simulink library "roller485lib"  (R2023a)
settings: Solver=VariableStepAuto  StartTime=0.0  StopTime=10.0  RelTol=1e-3
libraries: arduinolib x173, simulink x66
(part 1 of 6)
settings Model: Creator=kawata  LastModifiedBy=kawata
settings RTWCC: GPUComputeCapability=5.0

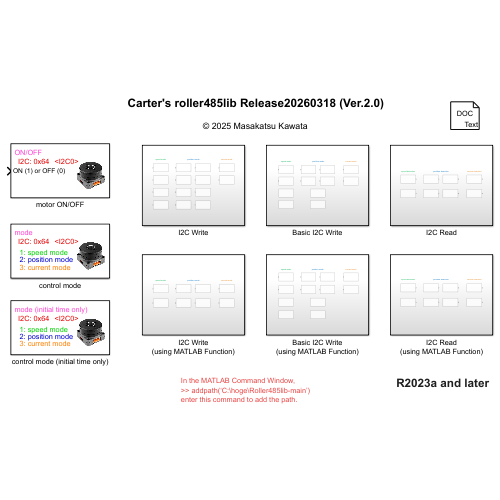
[thumbnail: Simulink's stored preview of the top-level diagram]
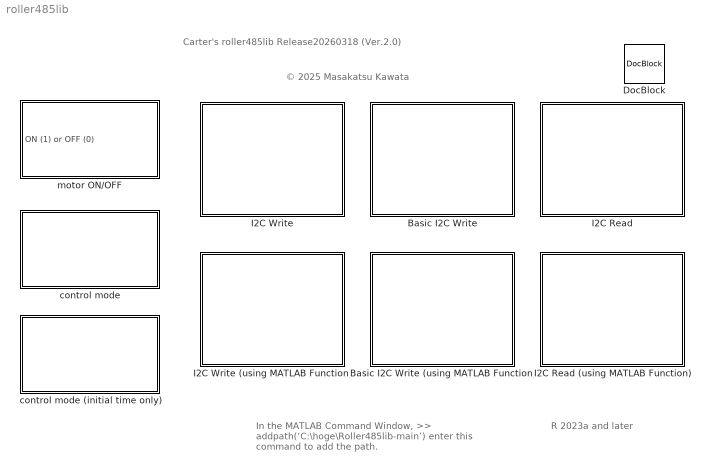
== system roller485lib ==
  note: © 2025 Masakatsu Kawata
  note: Carter's roller485lib Release20260318 (Ver.2.0)
  note: R 2023a and later
  note: In the MATLAB Command Window,
      | >> addpath(‘C:\hoge\Roller485lib-main’)
      | enter this command to add the path.
  Basic I2C Write : Subsystem
  Basic I2C Write (using MATLAB Function) : Subsystem
  DocBlock : simulink/Model-Wide Utilities/DocBlock  DocumentType=Text
      content=|
      | Carter's Roller485lib Ver.1.0
      | Copyright (c) 2025 Masakatsu Kawata
      | Released under the MIT License.
      | See LICENSE for details.
  I2C Read : Subsystem
  I2C Read (using MATLAB Function) : Subsystem
  I2C Write : Subsystem
  I2C Write (using MATLAB Function) : Subsystem
  control mode : Subsystem  mask{I2CAddress=0x64, I2CModule=0, control_mode=1}
      mask prompts: I2CAddress "I2C Address"; I2CModule "I2C Module"; control_mode "mode"
      mask help:
      | 1: speed mode (default)
      | 2: position mode
      | 3: current mode
      | 4: encoder mode
      mask TypeOptions I2CModule:
      | I2C Write
      | (0x01)/I2CModule
      mask DialogControl ParameterGroupVar Prompt: パラメーター
      mask Display:
      | image('roller485.png', [55,10,75,56]);
      | color('magenta');
      | text(5, 62, 'mode');
      | color('green');
      | text(12, 35, '1: speed mode');
      | color('blue');
      | text(12, 25, '2: position mode');
      | color('orange');
      | text(12, 15, '3: current mode');
      | 
      | color('red');
      | addr = get_param(gcb, 'I2CAddress');
      | text(10, 50, ['I2C: ' addr]);
      | 
      | color('red');
      | module = get_param(gcb, 'I2CModule');
      | text(60, 50, ['<I2C' module '>']);
  control mode (initial time only) : Subsystem  mask{I2CAddress=0x64, I2CModule=0, control_mode=1}
      mask prompts: I2CAddress "I2C Address"; I2CModule "I2C Module"; control_mode "mode"
      mask help:
      | 1: speed mode (default)
      | 2: position mode
      | 3: current mode
      | 4: encoder mode
      | ---------------------------------
      | valid only at the initial time
      mask TypeOptions I2CModule:
      | Enabled Subsystem/I2C Write
      | (0x01)/I2CModule
      mask DialogControl ParameterGroupVar Prompt: パラメーター
      mask Display:
      | image('roller485.png', [55,10,75,56]);
      | color('magenta');
      | text(5, 62, 'mode (initial time only)');
      | color('green');
      | text(12, 35, '1: speed mode');
      | color('blue');
      | text(12, 25, '2: position mode');
      | color('orange');
      | text(12, 15, '3: current mode');
      | 
      | color('red');
      | addr = get_param(gcb, 'I2CAddress');
      | text(10, 50, ['I2C: ' addr]);
      | 
      | color('red');
      | module = get_param(gcb, 'I2CModule');
      | text(60, 50, ['<I2C' module '>']);
  motor ON/OFF : Subsystem  mask{I2CAddress=0x64, I2CModule=0}
      mask prompts: I2CAddress "I2C Address"; I2CModule "I2C Module"
      mask help:
      | 0: motor off
      | 1: motor on
      mask TypeOptions I2CModule:
      | I2C Write
      | (0x00)/I2CModule
      mask DialogControl ParameterGroupVar Prompt: パラメーター
      mask Display:
      | image('roller485.png', [55,10,75,56]);
      | color('magenta');
      | text(5, 62, 'ON/OFF');
      | 
      | color('red');
      | addr = get_param(gcb, 'I2CAddress');
      | text(10, 50, ['I2C: ' addr]);
      | 
      | color('red');
      | module = get_param(gcb, 'I2CModule');
      | text(60, 50, ['<I2C' module '>']);

== system roller485lib/Basic I2C Write ==
  note: speed mode
  note: current mode
  note: position mode
  basic absolute angle command [deg] : Subsystem  mask{I2CAddress=0x64}
      mask prompts: I2CAddress "I2C Address"
      mask DialogControl ParameterGroupVar Prompt: パラメーター
      mask Display:
      | image('roller485.png', [55,10,75,56]);
      | color('blue');
      | text(10, 60, 'absolute position control');
      | 
      | color('red');
      | addr = get_param(gcb, 'I2CAddress');
      | text(17, 48, ['I2C: ' addr]);
  basic absolute angle command [rad] : Subsystem  mask{I2CAddress=0x64}
      mask prompts: I2CAddress "I2C Address"
      mask DialogControl ParameterGroupVar Prompt: パラメーター
      mask Display:
      | image('roller485.png', [55,10,75,56]);
      | color('blue');
      | text(10, 60, 'absolute position control');
      | 
      | color('red');
      | addr = get_param(gcb, 'I2CAddress');
      | text(17, 48, ['I2C: ' addr]);
  basic angular velocity command [rad/s] : Subsystem  mask{I2CAddress=0x64}
      mask prompts: I2CAddress "I2C Address"
      mask DialogControl ParameterGroupVar Prompt: パラメーター
      mask Display:
      | image('roller485.png', [55,10,75,56]);
      | color('green');
      | text(10, 60, 'speed control');
      | 
      | color('red');
      | addr = get_param(gcb, 'I2CAddress');
      | text(17, 48, ['I2C: ' addr]);
  basic angular velocity command [rpm] : Subsystem  mask{I2CAddress=0x64}
      mask prompts: I2CAddress "I2C Address"
      mask DialogControl ParameterGroupVar Prompt: パラメーター
      mask Display:
      | image('roller485.png', [55,10,75,56]);
      | color('green');
      | text(10, 60, 'speed control');
      | 
      | color('red');
      | addr = get_param(gcb, 'I2CAddress');
      | text(17, 48, ['I2C: ' addr]);
  basic current command [A] : Subsystem  mask{I2CAddress=0x64}
      mask prompts: I2CAddress "I2C Address"
      mask DialogControl ParameterGroupVar Prompt: パラメーター
      mask Display:
      | image('roller485.png', [55,10,75,56]);
      | color('orange');
      | text(10, 60, 'current control');
      | 
      | color('red');
      | addr = get_param(gcb, 'I2CAddress');
      | text(17, 48, ['I2C: ' addr]);
  basic current command [mA] : Subsystem  mask{I2CAddress=0x64}
      mask prompts: I2CAddress "I2C Address"
      mask DialogControl ParameterGroupVar Prompt: パラメーター
      mask Display:
      | image('roller485.png', [55,10,75,56]);
      | color('orange');
      | text(10, 60, 'current control');
      | 
      | color('red');
      | addr = get_param(gcb, 'I2CAddress');
      | text(17, 48, ['I2C: ' addr]);
  basic relative angle command [deg] : Subsystem  mask{I2CAddress=0x64, sample_time=-1}
      mask prompts: I2CAddress "I2C Address"; sample_time "Sample Time (-1 for inherited)"
      mask DialogControl ParameterGroupVar Prompt: パラメーター
      mask Display:
      | image('roller485.png', [55,10,75,56]);
      | color('blue');
      | text(10, 60, 'relative position control');
      | 
      | color('red');
      | addr = get_param(gcb, 'I2CAddress');
      | text(17, 48, ['I2C: ' addr]);
  basic relative angle command [rad] : Subsystem  mask{I2CAddress=0x64, sample_time=-1}
      mask prompts: I2CAddress "I2C Address"; sample_time "Sample Time (-1 for inherited)"
      mask DialogControl ParameterGroupVar Prompt: パラメーター
      mask Display:
      | image('roller485.png', [55,10,75,56]);
      | color('blue');
      | text(10, 60, 'relative position control');
      | 
      | color('red');
      | addr = get_param(gcb, 'I2CAddress');
      | text(17, 48, ['I2C: ' addr]);
  position PID : Subsystem  mask{I2CAddress=0x64, position_P=15, position_I=0.000003, position_D=400}
      mask prompts: I2CAddress "I2C Address"; position_P "P"; position_I "I"; position_D "D"
      mask help:
      | position mode
      | ---------------------------------
      | default value
      |  P: 15
      |  I: 0.000003
      |  D: 400
      mask DialogControl ParameterGroupVar Prompt: パラメーター
      mask Display:
      | image('roller485.png', [55,10,75,56]);
      | color('blue');
      | text(10, 60, 'position PID');
      | 
      | color('red');
      | addr = get_param(gcb, 'I2CAddress');
      | text(17, 48, ['I2C: ' addr]);
  position PID (within set time) : Subsystem  mask{I2CAddress=0x64, set_time=0, position_P=15, position_I=0.000003, position_D=400}
      mask prompts: I2CAddress "I2C Address"; set_time "Set Time"; position_P "P"; position_I "I"; position_D "D"
      mask help:
      | position mode
      | ---------------------------------
      | default value
      |  P: 15
      |  I: 0.000003
      |  D: 400
      | ---------------------------------
      | If t ≤ set_time, then PID gain can be set.
      mask DialogControl ParameterGroupVar Prompt: パラメーター
      mask Display:
      | image('roller485.png', [55,10,75,56]);
      | color('blue');
      | text(10, 60, 'position PID');
      | text(10, 47, '(within set time)');
      | 
      | color('red');
      | addr = get_param(gcb, 'I2CAddress');
      | text(17, 34, ['I2C: ' addr]);
  speed PID : Subsystem  mask{I2CAddress=0x64, speed_P=15, speed_I=0.0001, speed_D=400}
      mask prompts: I2CAddress "I2C Address"; speed_P "P"; speed_I "I"; speed_D "D"
      mask help:
      | speed mode
      | ---------------------------------
      | default value (PID gain of speed controller)
      |      P: 15,  I: 0.0001,  D: 400
      | recommended value (PID gain of speed controller)
      |      P: 2,  I: 0,  D: 850
      mask DialogControl ParameterGroupVar Prompt: パラメーター
      mask Display:
      | image('roller485.png', [55,10,75,56]);
      | color('green');
      | text(10, 60, 'speed PID');
      | 
      | color('red');
      | addr = get_param(gcb, 'I2CAddress');
      | text(17, 48, ['I2C: ' addr]);
  speed PID (within set time) : Subsystem  mask{I2CAddress=0x64, set_time=0, speed_P=15, speed_I=0.0001, speed_D=400}
      mask prompts: I2CAddress "I2C Address"; set_time "Set Time"; speed_P "P"; speed_I "I"; speed_D "D"
      mask help:
      | speed mode
      | ---------------------------------
      | default value (PID gain of speed controller)
      |      P: 15,  I: 0.0001,  D: 400
      | recommended value (PID gain of speed controller)
      |      P: 2,  I: 0,  D: 850
      | ---------------------------------
      | valid only at the initial time
      | ---------------------------------
      | If t ≤ set_time, then PID gain can be set.
      mask DialogControl ParameterGroupVar Prompt: パラメーター
      mask Display:
      | image('roller485.png', [55,10,75,56]);
      | color('green');
      | text(10, 60, 'speed PID');
      | text(10, 47, '(within set time)');
      | 
      | color('red');
      | addr = get_param(gcb, 'I2CAddress');
      | text(17, 34, ['I2C: ' addr]);

== system roller485lib/Basic I2C Write (using MATLAB Function) ==
  note: position mode
  note: current mode
  note: speed mode
  basic absolute angle command [deg] (using MATLAB Function) : Subsystem  mask{I2CAddress=0x64}
      mask prompts: I2CAddress "I2C Address"
      mask DialogControl ParameterGroupVar Prompt: パラメーター
      mask Display:
      | image('roller485_matlab_fcn.png', [55,10,75,56]);
      | color('blue');
      | text(10, 60, 'absolute position control');
      | 
      | color('red');
      | addr = get_param(gcb, 'I2CAddress');
      | text(17, 48, ['I2C: ' addr]);
  basic absolute angle command [rad] (using MATLAB Function) : Subsystem  mask{I2CAddress=0x64}
      mask prompts: I2CAddress "I2C Address"
      mask DialogControl ParameterGroupVar Prompt: パラメーター
      mask Display:
      | image('roller485_matlab_fcn.png', [55,10,75,56]);
      | color('blue');
      | text(10, 60, 'absolute position control');
      | 
      | color('red');
      | addr = get_param(gcb, 'I2CAddress');
      | text(17, 48, ['I2C: ' addr]);
  basic angular velocity command [rad/s] (using MATLAB Function) : Subsystem  mask{I2CAddress=0x64}
      mask prompts: I2CAddress "I2C Address"
      mask DialogControl ParameterGroupVar Prompt: パラメーター
      mask Display:
      | image('roller485_matlab_fcn.png', [55,10,75,56]);
      | color('green');
      | text(10, 60, 'speed control');
      | 
      | color('red');
      | addr = get_param(gcb, 'I2CAddress');
      | text(17, 48, ['I2C: ' addr]);
  basic angular velocity command [rpm] (using MATLAB Function) : Subsystem  mask{I2CAddress=0x64}
      mask prompts: I2CAddress "I2C Address"
      mask DialogControl ParameterGroupVar Prompt: パラメーター
      mask Display:
      | image('roller485_matlab_fcn.png', [55,10,75,56]);
      | color('green');
      | text(10, 60, 'speed control');
      | 
      | color('red');
      | addr = get_param(gcb, 'I2CAddress');
      | text(17, 48, ['I2C: ' addr]);
  basic current command [A] (using MATLAB Function) : Subsystem  mask{I2CAddress=0x64}
      mask prompts: I2CAddress "I2C Address"
      mask DialogControl ParameterGroupVar Prompt: パラメーター
      mask Display:
      | image('roller485_matlab_fcn.png', [55,10,75,56]);
      | color('orange');
      | text(10, 60, 'current control');
      | 
      | color('red');
      | addr = get_param(gcb, 'I2CAddress');
      | text(17, 48, ['I2C: ' addr]);
  basic current command [mA] (using MATLAB Function) : Subsystem  mask{I2CAddress=0x64}
      mask prompts: I2CAddress "I2C Address"
      mask DialogControl ParameterGroupVar Prompt: パラメーター
      mask Display:
      | image('roller485_matlab_fcn.png', [55,10,75,56]);
      | color('orange');
      | text(10, 60, 'current control');
      | 
      | color('red');
      | addr = get_param(gcb, 'I2CAddress');
      | text(17, 48, ['I2C: ' addr]);
  basic relative angle command [deg] (using MATLAB Function) : Subsystem  mask{I2CAddress=0x64, sample_time=-1}
      mask prompts: I2CAddress "I2C Address"; sample_time "Sample Time (-1 for inherited)"
      mask DialogControl ParameterGroupVar Prompt: パラメーター
      mask Display:
      | image('roller485_matlab_fcn.png', [55,10,75,56]);
      | color('blue');
      | text(10, 60, 'relative position control');
      | 
      | color('red');
      | addr = get_param(gcb, 'I2CAddress');
      | text(17, 48, ['I2C: ' addr]);
  basic relative angle command [rad] (using MATLAB Function) : Subsystem  mask{I2CAddress=0x64, sample_time=-1}
      mask prompts: I2CAddress "I2C Address"; sample_time "Sample Time (-1 for inherited)"
      mask DialogControl ParameterGroupVar Prompt: パラメーター
      mask Display:
      | image('roller485_matlab_fcn.png', [55,10,75,56]);
      | color('blue');
      | text(10, 60, 'relative position control');
      | 
      | color('red');
      | addr = get_param(gcb, 'I2CAddress');
      | text(17, 48, ['I2C: ' addr]);
  position PID (using MATLAB Function) : Subsystem  mask{I2CAddress=0x64, position_P=15, position_I=0.000003, position_D=400}
      mask prompts: I2CAddress "I2C Address"; position_P "P"; position_I "I"; position_D "D"
      mask help:
      | position mode
      | ---------------------------------
      | default value
      |  P: 15
      |  I: 0.000003
      |  D: 400
      mask DialogControl ParameterGroupVar Prompt: パラメーター
      mask Display:
      | image('roller485_matlab_fcn.png', [55,10,75,56]);
      | color('blue');
      | text(10, 60, 'position PID');
      | 
      | color('red');
      | addr = get_param(gcb, 'I2CAddress');
      | text(17, 48, ['I2C: ' addr]);
  position PID (within set time) (using MATLAB Function) : Subsystem  mask{I2CAddress=0x64, set_time=0, position_P=15, position_I=0.000003, position_D=400}
      mask prompts: I2CAddress "I2C Address"; set_time "Set Time"; position_P "P"; position_I "I"; position_D "D"
      mask help:
      | position mode
      | ---------------------------------
      | default value
      |  P: 15
      |  I: 0.000003
      |  D: 400
      | ---------------------------------
      | If t ≤ set_time, then PID gain can be set.
      mask DialogControl ParameterGroupVar Prompt: パラメーター
      mask Display:
      | image('roller485_matlab_fcn.png', [55,10,75,56]);
      | color('blue');
      | text(10, 60, 'position PID');
      | text(10, 47, '(within set time)');
      | 
      | color('red');
      | addr = get_param(gcb, 'I2CAddress');
      | text(17, 34, ['I2C: ' addr]);
  speed PID (using MATLAB Function) : Subsystem  mask{I2CAddress=0x64, speed_P=15, speed_I=0.0001, speed_D=400}
      mask prompts: I2CAddress "I2C Address"; speed_P "P"; speed_I "I"; speed_D "D"
      mask help:
      | speed mode
      | ---------------------------------
      | default value (PID gain of speed controller)
      |      P: 15,  I: 0.0001,  D: 400
      | recommended value (PID gain of speed controller)
      |      P: 2,  I: 0,  D: 850
      mask DialogControl ParameterGroupVar Prompt: パラメーター
      mask Display:
      | image('roller485_matlab_fcn.png', [55,10,75,56]);
      | color('green');
      | text(10, 60, 'speed PID');
      | 
      | color('red');
      | addr = get_param(gcb, 'I2CAddress');
      | text(17, 48, ['I2C: ' addr]);
  speed PID (within set time) (using MATLAB Function) : Subsystem  mask{I2CAddress=0x64, set_time=0, speed_P=15, speed_I=0.0001, speed_D=400}
      mask prompts: I2CAddress "I2C Address"; set_time "Set Time"; speed_P "P"; speed_I "I"; speed_D "D"
      mask help:
      | speed mode
      | ---------------------------------
      | default value (PID gain of speed controller)
      |      P: 15,  I: 0.0001,  D: 400
      | recommended value (PID gain of speed controller)
      |      P: 2,  I: 0,  D: 850
      | ---------------------------------
      | If t ≤ set_time, then PID gain can be set.
      mask DialogControl ParameterGroupVar Prompt: パラメーター
      mask Display:
      | image('roller485_matlab_fcn.png', [55,10,75,56]);
      | color('green');
      | text(10, 60, 'speed PID');
      | text(10, 47, '(within set time)');
      | 
      | color('red');
      | addr = get_param(gcb, 'I2CAddress');
      | text(17, 34, ['I2C: ' addr]);

== system roller485lib/I2C Read ==
  note: speed detection
  note: current detection
  note: position detection
  absolute angle detection [deg] : Subsystem  mask{I2CAddress=0x64, I2CModule=0, sample_time=-1}
      mask prompts: I2CAddress "I2C Address"; I2CModule "I2C Module"; sample_time "Sample Time (-1 for inherited)"
      mask TypeOptions I2CModule:
      | I2C Read
      | (0x90)/I2CModule
      mask DialogControl ParameterGroupVar Prompt: パラメーター
      mask Display:
      | image('roller485.png', [30,10,75,56]);
      | color('blue');
      | text(5, 62, 'absolute angle detection');
      | 
      | color('red');
      | addr = get_param(gcb, 'I2CAddress');
      | text(10, 50, ['I2C: ' addr]);
      | 
      | color('red');
      | module = get_param(gcb, 'I2CModule');
      | text(10, 40, ['<I2C' module '>']);
  absolute angle detection [rad] : Subsystem  mask{I2CAddress=0x64, I2CModule=0, sample_time=-1}
      mask prompts: I2CAddress "I2C Address"; I2CModule "I2C Module"; sample_time "Sample Time (-1 for inherited)"
      mask TypeOptions I2CModule:
      | I2C Read
      | (0x90)/I2CModule
      mask DialogControl ParameterGroupVar Prompt: パラメーター
      mask Display:
      | image('roller485.png', [30,10,75,56]);
      | 
      | color('blue');
      | text(5, 62, 'absolute angle detection');
      | 
      | color('red');
      | addr = get_param(gcb, 'I2CAddress');
      | text(10, 50, ['I2C: ' addr]);
      | 
      | color('red');
      | module = get_param(gcb, 'I2CModule');
      | text(10, 40, ['<I2C' module '>']);
  angular velocity detection using LPF [rad/s] : Subsystem  mask{I2CAddress=0x64, I2CModule=0, sample_time=-1}
      mask prompts: I2CAddress "I2C Address"; I2CModule "I2C Module"; sample_time "Sample Time (-1 for inherited)"
      mask TypeOptions I2CModule:
      | I2C Read
      | (0x60)/I2CModule
      mask DialogControl ParameterGroupVar Prompt: パラメーター
      mask Display:
      | image('roller485.png', [30,10,75,56]);
      | color('green');
      | text(5, 62, 'speed detection');
      | 
      | color('red');
      | addr = get_param(gcb, 'I2CAddress');
      | text(10, 50, ['I2C: ' addr]);
      | 
      | color('red');
      | module = get_param(gcb, 'I2CModule');
      | text(10, 40, ['<I2C' module '>']);
  angular velocity detection using LPF [rpm] : Subsystem  mask{I2CAddress=0x64, I2CModule=0, sample_time=-1}
      mask prompts: I2CAddress "I2C Address"; I2CModule "I2C Module"; sample_time "Sample Time (-1 for inherited)"
      mask TypeOptions I2CModule:
      | I2C Read
      | (0x60)/I2CModule
      mask DialogControl ParameterGroupVar Prompt: パラメーター
      mask Display:
      | image('roller485.png', [30,10,75,56]);
      | color('green');
      | text(5, 62, 'speed detection');
      | 
      | color('red');
      | addr = get_param(gcb, 'I2CAddress');
      | text(10, 50, ['I2C: ' addr]);
      | 
      | color('red');
      | module = get_param(gcb, 'I2CModule');
      | text(10, 40, ['<I2C' module '>']);
  current detection [A] : Subsystem  mask{I2CAddress=0x64, I2CModule=0, sample_time=-1}
      mask prompts: I2CAddress "I2C Address"; I2CModule "I2C Module"; sample_time "Sample Time (-1 for inherited)"
      mask TypeOptions I2CModule:
      | I2C Read
      | (0xC0)/I2CModule
      mask DialogControl ParameterGroupVar Prompt: パラメーター
      mask Display:
      | image('roller485.png', [30,10,75,56]);
      | color('orange');
      | text(5, 62, 'current detection');
      | 
      | color('red');
      | addr = get_param(gcb, 'I2CAddress');
      | text(10, 50, ['I2C: ' addr]);
      | 
      | color('red');
      | module = get_param(gcb, 'I2CModule');
      | text(10, 40, ['<I2C' module '>']);
  current detection [mA] : Subsystem  mask{I2CAddress=0x64, I2CModule=0, sample_time=-1}
      mask prompts: I2CAddress "I2C Address"; I2CModule "I2C Module"; sample_time "Sample Time (-1 for inherited)"
      mask TypeOptions I2CModule:
      | I2C Read
      | (0xC0)/I2CModule
      mask DialogControl ParameterGroupVar Prompt: パラメーター
      mask Display:
      | image('roller485.png', [30,10,75,56]);
      | 
      | color('orange');
      | text(5, 62, 'current detection');
      | 
      | color('red');
      | addr = get_param(gcb, 'I2CAddress');
      | text(10, 50, ['I2C: ' addr]);
      | 
      | color('red');
      | module = get_param(gcb, 'I2CModule');
      | text(10, 40, ['<I2C' module '>']);
  relative angle detection [deg] : Subsystem  mask{I2CAddress=0x64, I2CModule=0, sample_time=-1, set_time=0}
      mask prompts: I2CAddress "I2C Address"; I2CModule "I2C Module"; sample_time "Sample Time (-1 for inherited)"; set_time "Set Time"
      mask help: If t ≤ set_time, then initial angle is set.
      mask TypeOptions I2CModule:
      | I2C Read
      | (0x90)/I2CModule
      mask DialogControl ParameterGroupVar Prompt: パラメーター
      mask Display:
      | image('roller485.png', [30,10,75,56]);
      | 
      | color('blue');
      | text(5, 62, 'relative angle detection');
      | 
      | color('red');
      | addr = get_param(gcb, 'I2CAddress');
      | text(10, 50, ['I2C: ' addr]);
      | 
      | color('red');
      | module = get_param(gcb, 'I2CModule');
      | text(10, 40, ['<I2C' module '>']);
  relative angle detection [rad] : Subsystem  mask{I2CAddress=0x64, I2CModule=0, sample_time=-1, set_time=0}
      mask prompts: I2CAddress "I2C Address"; I2CModule "I2C Module"; sample_time "Sample Time (-1 for inherited)"; set_time "Set Time"
      mask help: If t ≤ set_time, then initial angle is set.
      mask TypeOptions I2CModule:
      | I2C Read
      | (0x90)/I2CModule
      mask DialogControl ParameterGroupVar Prompt: パラメーター
      mask Display:
      | image('roller485.png', [30,10,75,56]);
      | 
      | color('blue');
      | text(5, 62, 'relative angle detection');
      | 
      | color('red');
      | addr = get_param(gcb, 'I2CAddress');
      | text(10, 50, ['I2C: ' addr]);
      | 
      | color('red');
      | module = get_param(gcb, 'I2CModule');
      | text(10, 40, ['<I2C' module '>']);

== system roller485lib/I2C Read (using MATLAB Function) ==
  note: position detection
  note: current detection
  note: speed detection
  absolute angle detection [deg] (using MATLAB Function) : Subsystem  mask{I2CAddress=0x64, I2CModule=0, sample_time=-1}
      mask prompts: I2CAddress "I2C Address"; I2CModule "I2C Module"; sample_time "Sample Time (-1 for inherited)"
      mask TypeOptions I2CModule:
      | I2C Read
      | (0x90)/I2CModule
      mask DialogControl ParameterGroupVar Prompt: パラメーター
      mask Display:
      | image('roller485_matlab_fcn.png', [38,10,75,56]);
      | 
      | color('blue');
      | text(5, 62, 'absolute angle detection');
      | 
      | color('red');
      | addr = get_param(gcb, 'I2CAddress');
      | text(10, 50, ['I2C: ' addr]);
      | 
      | color('red');
      | module = get_param(gcb, 'I2CModule');
      | text(10, 40, ['<I2C' module '>']);
  absolute angle detection [rad] (using MATLAB Function) : Subsystem  mask{I2CAddress=0x64, I2CModule=0, sample_time=-1}
      mask prompts: I2CAddress "I2C Address"; I2CModule "I2C Module"; sample_time "Sample Time (-1 for inherited)"
      mask TypeOptions I2CModule:
      | I2C Read
      | (0x90)/I2CModule
      mask DialogControl ParameterGroupVar Prompt: パラメーター
      mask Display:
      | image('roller485_matlab_fcn.png', [38,10,75,56]);
      | 
      | color('blue');
      | text(5, 62, 'absolute angle detection');
      | 
      | color('red');
      | addr = get_param(gcb, 'I2CAddress');
      | text(10, 50, ['I2C: ' addr]);
      | 
      | color('red');
      | module = get_param(gcb, 'I2CModule');
      | text(10, 40, ['<I2C' module '>']);
  angular velocity detection using LPF [rad/s] (using MATLAB Function) : Subsystem  mask{I2CAddress=0x64, I2CModule=0, sample_time=-1}
      mask prompts: I2CAddress "I2C Address"; I2CModule "I2C Module"; sample_time "Sample Time (-1 for inherited)"
      mask TypeOptions I2CModule:
      | I2C Read
      | (0x60)/I2CModule
      mask DialogControl ParameterGroupVar Prompt: パラメーター
      mask Display:
      | image('roller485_matlab_fcn.png', [38,10,75,56]);
      | 
      | color('green');
      | text(5, 62, 'speed detection');
      | 
      | color('red');
      | addr = get_param(gcb, 'I2CAddress');
      | text(10, 50, ['I2C: ' addr]);
      | 
      | color('red');
      | module = get_param(gcb, 'I2CModule');
      | text(10, 40, ['<I2C' module '>']);
  angular velocity detection using LPF [rpm] (using MATLAB Function) : Subsystem  mask{I2CAddress=0x64, I2CModule=0, sample_time=-1}
      mask prompts: I2CAddress "I2C Address"; I2CModule "I2C Module"; sample_time "Sample Time (-1 for inherited)"
      mask TypeOptions I2CModule:
      | I2C Read
      | (0x60)/I2CModule
      mask DialogControl ParameterGroupVar Prompt: パラメーター
      mask Display:
      | image('roller485_matlab_fcn.png', [38,10,75,56]);
      | 
      | color('green');
      | text(5, 62, 'speed detection');
      | 
      | color('red');
      | addr = get_param(gcb, 'I2CAddress');
      | text(10, 50, ['I2C: ' addr]);
      | 
      | color('red');
      | module = get_param(gcb, 'I2CModule');
      | text(10, 40, ['<I2C' module '>']);
  current detection [A] (using MATLAB Function) : Subsystem  mask{I2CAddress=0x64, I2CModule=0, sample_time=-1}
      mask prompts: I2CAddress "I2C Address"; I2CModule "I2C Module"; sample_time "Sample Time (-1 for inherited)"
      mask TypeOptions I2CModule:
      | I2C Read
      | (0xC0)/I2CModule
      mask DialogControl ParameterGroupVar Prompt: パラメーター
      mask Display:
      | image('roller485_matlab_fcn.png', [38,10,75,56]);
      | 
      | color('orange');
      | text(5, 62, 'current detection');
      | 
      | color('red');
      | addr = get_param(gcb, 'I2CAddress');
      | text(10, 50, ['I2C: ' addr]);
      | 
      | color('red');
      | module = get_param(gcb, 'I2CModule');
      | text(10, 40, ['<I2C' module '>']);
  current detection [mA] (using MATLAB Function) : Subsystem  mask{I2CAddress=0x64, I2CModule=0, sample_time=-1}
      mask prompts: I2CAddress "I2C Address"; I2CModule "I2C Module"; sample_time "Sample Time (-1 for inherited)"
      mask TypeOptions I2CModule:
      | I2C Read
      | (0xC0)/I2CModule
      mask DialogControl ParameterGroupVar Prompt: パラメーター
      mask Display:
      | image('roller485_matlab_fcn.png', [38,10,75,56]);
      | 
      | color('orange');
      | text(5, 62, 'current detection');
      | 
      | color('red');
      | addr = get_param(gcb, 'I2CAddress');
      | text(10, 50, ['I2C: ' addr]);
      | 
      | color('red');
      | module = get_param(gcb, 'I2CModule');
      | text(10, 40, ['<I2C' module '>']);
  relative angle detection [deg] (using MATLAB Function) : Subsystem  mask{I2CAddress=0x64, I2CModule=0, sample_time=-1, set_time=0}
      mask prompts: I2CAddress "I2C Address"; I2CModule "I2C Module"; sample_time "Sample Time (-1 for inherited)"; set_time "Set Time"
      mask help: If t ≤ set_time, then initial angle is set.
      mask TypeOptions I2CModule:
      | I2C Read
      | (0x90)/I2CModule
      mask DialogControl ParameterGroupVar Prompt: パラメーター
      mask Display:
      | image('roller485_matlab_fcn.png', [38,10,75,56]);
      | 
      | color('blue');
      | text(5, 62, 'relative angle detection');
      | 
      | color('red');
      | addr = get_param(gcb, 'I2CAddress');
      | text(10, 50, ['I2C: ' addr]);
      | 
      | color('red');
      | module = get_param(gcb, 'I2CModule');
      | text(10, 40, ['<I2C' module '>']);
  relative angle detection [rad] (using MATLAB Function) : Subsystem  mask{I2CAddress=0x64, I2CModule=0, sample_time=-1, set_time=0}
      mask prompts: I2CAddress "I2C Address"; I2CModule "I2C Module"; sample_time "Sample Time (-1 for inherited)"; set_time "Set Time"
      mask help: If t ≤ set_time, then initial angle is set.
      mask TypeOptions I2CModule:
      | I2C Read
      | (0x90)/I2CModule
      mask DialogControl ParameterGroupVar Prompt: パラメーター
      mask Display:
      | image('roller485_matlab_fcn.png', [38,10,75,56]);
      | 
      | color('blue');
      | text(5, 62, 'relative angle detection');
      | 
      | color('red');
      | addr = get_param(gcb, 'I2CAddress');
      | text(10, 50, ['I2C: ' addr]);
      | 
      | color('red');
      | module = get_param(gcb, 'I2CModule');
      | text(10, 40, ['<I2C' module '>']);
